simulink model "Pendulo_invertido"  (R2025b)
settings: Solver=VariableStepAuto  StartTime=0.0  StopTime=10.0  RelTol=1e-3
values from neighbouring files (symbols this model uses):
  Beq = 0.25    [Pendulo_Invertido.m]    (also in Pendulo_invertido.mat = 4.3)
  Bp = 0.2    [Pendulo_Invertido.m]    (also in Pendulo_invertido.mat = 0.0024)
  Fc = 0    [Pendulo_invertido.mat]
  g = 9.81    [Pendulo_Invertido.m]    (also in Pendulo_invertido.mat)
  Ip = 0.2    [Pendulo_Invertido.m]    (also in Pendulo_invertido.mat = 0.0079)
  lp = 0.3    [Pendulo_Invertido.m]    (also in Pendulo_invertido.mat = 0.3302)
  Mc = 0.2    [Pendulo_Invertido.m]    (also in Pendulo_invertido.mat = 0.7031)
  Mp = 0.1    [Pendulo_Invertido.m]    (also in Pendulo_invertido.mat = 0.23)
settings Model: Creator=Diego  LastModifiedBy=Diego

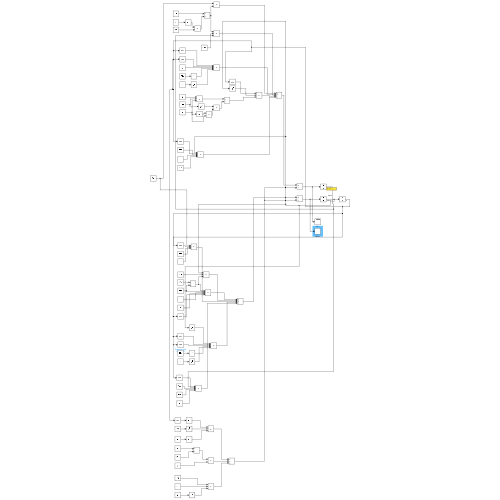
[thumbnail: Simulink's stored preview of the top-level diagram]
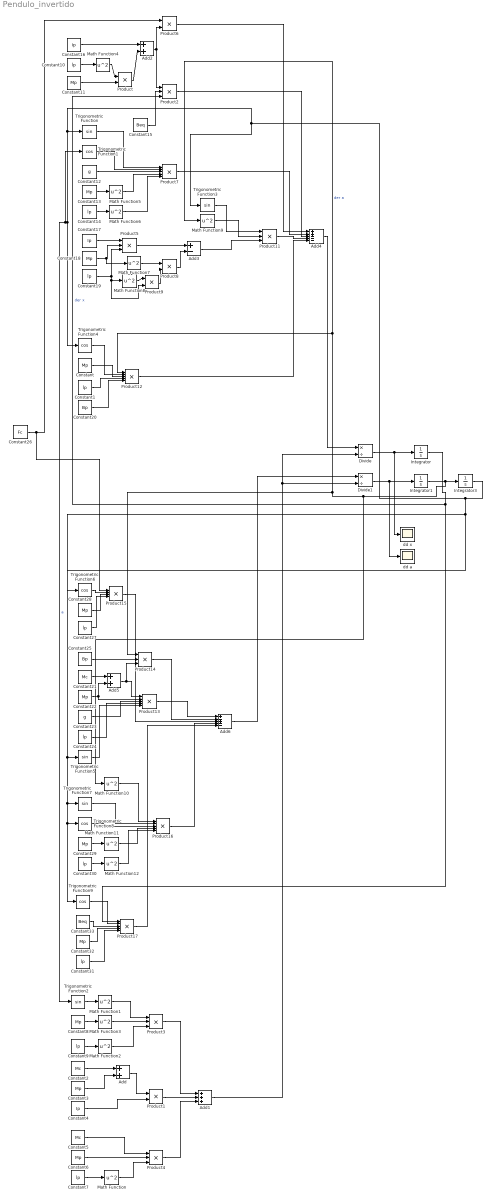
== system Pendulo_invertido ==
  Add : Sum
  Add1 : Sum  Inputs=+++
  Add2 : Sum
  Add3 : Sum  Inputs=+-
  Add4 : Sum  Inputs=++---
  Add5 : Sum
  Add6 : Sum  Inputs=+-+--
  Constant{,3,6,8,11,13,18,22,28..29,32} (11 alike) : Constant  Value=Mp
  Constant{1,7,9..10,14,19,24,27,30..31} (10 alike) : Constant  Value=lp
  Constant12 : Constant  Value=g
  Constant15 : Constant  Value=Beq
  Constant16 : Constant  Value=Ip
  Constant17 : Constant  Value=Ip
  Constant2 : Constant  Value=Mc
  Constant20 : Constant  Value=Bp
  Constant21 : Constant  Value=Mc
  Constant23 : Constant  Value=g
  Constant25 : Constant  Value=Bp
  Constant26 : Constant  Value=Fc
  Constant33 : Constant  Value=Beq
  Constant4 : Constant  Value=Ip
  Constant5 : Constant  Value=Mc
  Divide : Product  Inputs=*/
  Divide1 : Product  Inputs=*/
  Integrator : Integrator
  Integrator1 : Integrator
  Integrator3 : Integrator
  Math Function{,1..12} (13 alike) : Math  Operator=square
  Product{,1,6,8..9} (5 alike) : Product
  Product{2..5,11,14} (6 alike) : Product  Inputs=3
  Product{7,12..13,16..17} (5 alike) : Product  Inputs=5
  Product15 : Product  Inputs=4
  Trigonometric Function{,2..3,5,7} (5 alike) : Trigonometry
  Trigonometric Function{1,4,6,8..9} (5 alike) : Trigonometry  Operator=cos
  "dd a " : Scope
      settings: ActiveDisplayYMinimum=-1.0281643534245157  ActiveDisplayYMaximum=1.0308976029129711
  dd x : Scope
      settings: ActiveDisplayYMinimum=-21.720179733836122  ActiveDisplayYMaximum=21.314181231157825
  wires:
  Integrator3/1 -> Trigonometric Function6/1, Trigonometric Function9/1, Trigonometric Function8/1, Trigonometric Function7/1, Trigonometric Function5/1, Trigonometric Function4/1, Trigonometric Function2/1, Trigonometric Function1/1, Trigonometric Function/1, Trigonometric Function3/1  "a"
  Constant2/1 -> Add/1
  Constant3/1 -> Add/2
  Add/1 -> Product1/1
  Constant4/1 -> Product1/2
  Constant7/1 -> Math Function/1
  Trigonometric Function2/1 -> Math Function1/1
  Constant8/1 -> Math Function3/1
  Constant9/1 -> Math Function2/1
  Math Function2/1 -> Product3/3
  Math Function3/1 -> Product3/2
  Math Function1/1 -> Product3/1
  Product3/1 -> Add1/1
  Product1/1 -> Add1/2
  Product4/1 -> Add1/3
  Constant10/1 -> Math Function4/1
  Math Function4/1 -> Product/1
  Constant11/1 -> Product/2
  Product/1 -> Add2/2
  Constant26/1 -> Product15/1, Product6/1
  Add2/1 -> Product2/1, Product6/2
  Constant13/1 -> Math Function5/1
  Constant14/1 -> Math Function6/1
  Math Function/1 -> Product4/3
  Constant6/1 -> Product4/2
  Constant5/1 -> Product4/1
  Math Function6/1 -> Product7/5
  Math Function5/1 -> Product7/4
  Constant12/1 -> Product7/3
  Trigonometric Function1/1 -> Product7/2
  Trigonometric Function/1 -> Product7/1
  Constant15/1 -> Product2/2
  Constant16/1 -> Add2/1
  Constant17/1 -> Product5/1
  Constant18/1 -> Math Function7/1, Product5/2
  Constant19/1 -> Math Function8/1, Product9/2, Product5/3
  Math Function7/1 -> Product8/1
  Math Function8/1 -> Product9/1
  Product9/1 -> Product8/2
  Product5/1 -> Add3/1
  Product8/1 -> Add3/2
  Integrator/1 -> Product17/1, Product2/3  "der x"
  Integrator1/1 -> Math Function10/1, Product14/1, Math Function9/1, Product12/1, Integrator3/1  "der a"
  Math Function9/1 -> Product11/2
  Trigonometric Function3/1 -> Product11/1
  Constant20/1 -> Product12/5
  Constant1/1 -> Product12/4
  Constant/1 -> Product12/3
  Trigonometric Function4/1 -> Product12/2
  Product12/1 -> Add4/5
  Product11/1 -> Add4/4
  Product2/1 -> Add4/3
  Product7/1 -> Add4/2
  Product6/1 -> Add4/1
  Add4/1 -> Divide/1
  Add1/1 -> Divide1/2, Divide/2
  Divide/1 -> dd x/1, Integrator/1
  Constant21/1 -> Add5/1
  Constant22/1 -> Product13/2, Add5/2
  Add5/1 -> Product14/3, Product13/1
  Constant23/1 -> Product13/3
  Constant24/1 -> Product13/4
  Trigonometric Function5/1 -> Product13/5
  Constant25/1 -> Product14/2
  Trigonometric Function6/1 -> Product15/2
  Constant28/1 -> Product15/3
  Constant27/1 -> Product15/4
  Constant29/1 -> Math Function11/1
  Constant30/1 -> Math Function12/1
  Math Function10/1 -> Product16/1
  Trigonometric Function7/1 -> Product16/2
  Trigonometric Function8/1 -> Product16/3
  Math Function11/1 -> Product16/4
  Math Function12/1 -> Product16/5
  Constant31/1 -> Product17/5
  Constant32/1 -> Product17/4
  Constant33/1 -> Product17/3
  Trigonometric Function9/1 -> Product17/2
  Product13/1 -> Add6/1
  Product14/1 -> Add6/2
  Product15/1 -> Add6/3
  Product16/1 -> Add6/4
  Product17/1 -> Add6/5
  Divide1/1 -> "dd a "/1, Integrator1/1
  Add6/1 -> Divide1/1
  Add3/1 -> Product11/3
